simulink model "osservatore_con_fnc"  (R2024b)
settings: Solver=VariableStepAuto  StartTime=0.0  StopTime=10.0  RelTol=1e-3
values from neighbouring files (symbols this model uses):
  A4 = horzcat([0;0;0;0], A4)    [stabilita_AS.m]
  BB = [0; B]    [stabilita_AS.m]
  KK = [0 K]    [stabilita_AS.m]
undefined symbols (not defined in the file or in its folder): L_oss_theta
settings Model: Creator=costa  LastModifiedBy=costa

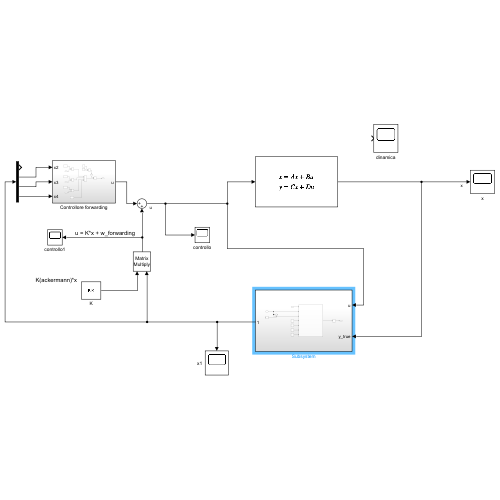
[thumbnail: Simulink's stored preview of the top-level diagram]
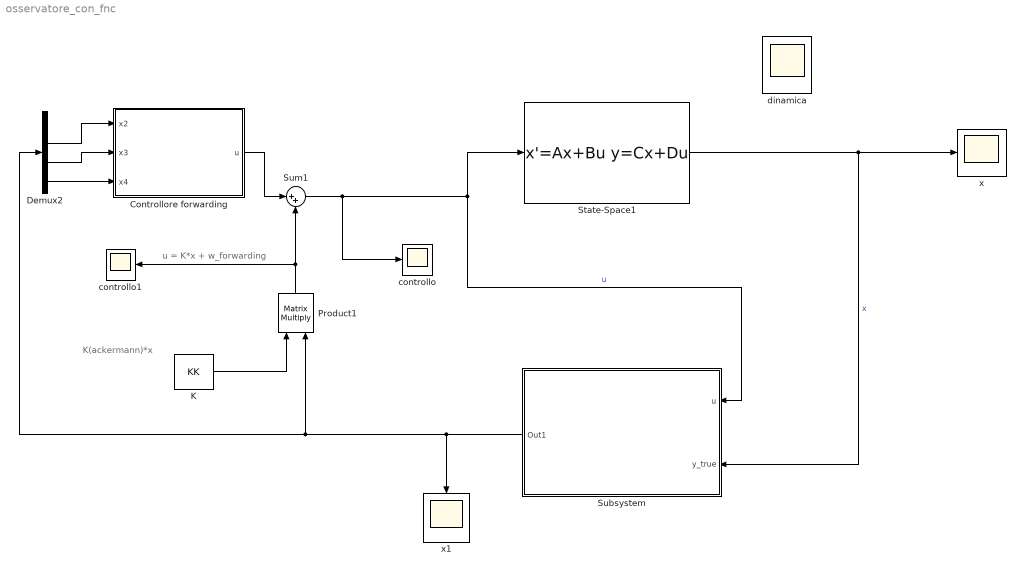
== system osservatore_con_fnc ==
  note: K(ackermann)*x
  note: u = K*x + w_forwarding
  Controllore forwarding : Subsystem
  Demux2 : Demux
  K : Constant  Value=KK  VectorParams1D=off
  Product1 : Product  Multiplication=Matrix(*)
  State-Space1 : StateSpace  A=A4  B=BB  C=eye(4)  D=[0; 0; 0; 0]  InitialCondition=[1 0 0 0]
  Subsystem : Subsystem
  Sum1 : Sum  Inputs=|++
  controllo : Scope
  controllo1 : Scope
  dinamica : Scope
  x : Scope
  x1 : Scope
  wires:
  K/1 -> Product1/1
  Sum1/1 -> controllo/1, State-Space1/1, Subsystem/1(u)  "u"
  State-Space1/1 -> Subsystem/2(y_true), x/1  "x"
  Product1/1 -> controllo1/1, Sum1/2
  Subsystem/1(Out1) -> Demux2/1, Product1/2, x1/1
  Demux2/2 -> Controllore forwarding/1(x2)
  Demux2/3 -> Controllore forwarding/2(x3)
  Demux2/4 -> Controllore forwarding/3(x4)
  Controllore forwarding/1(u) -> Sum1/1

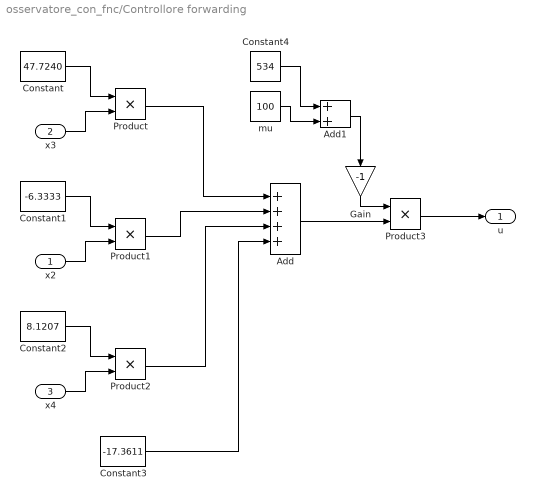
== system osservatore_con_fnc/Controllore forwarding ==
  x2 : Inport
  x3 : Inport  Port=2
  x4 : Inport  Port=3
  Add : Sum  Inputs=++++
  Add1 : Sum
  Constant : Constant  Value=47.7240
  Constant1 : Constant  Value=-6.3333
  Constant2 : Constant  Value=8.1207
  Constant3 : Constant  Value=-17.3611
  Constant4 : Constant  Value=534
  Gain : Gain  Gain=-1
  Product{,1..3} (4 alike) : Product
  mu : Constant  Value=100
  u : Outport
  wires:
  x3/1 -> Product/2
  Constant/1 -> Product/1
  Constant1/1 -> Product1/1
  x2/1 -> Product1/2
  Constant2/1 -> Product2/1
  x4/1 -> Product2/2
  Product/1 -> Add/1
  Product1/1 -> Add/2
  Product2/1 -> Add/3
  Constant3/1 -> Add/4
  Add/1 -> Product3/2
  Product3/1 -> u/1
  Constant4/1 -> Add1/1
  mu/1 -> Add1/2
  Add1/1 -> Gain/1
  Gain/1 -> Product3/1

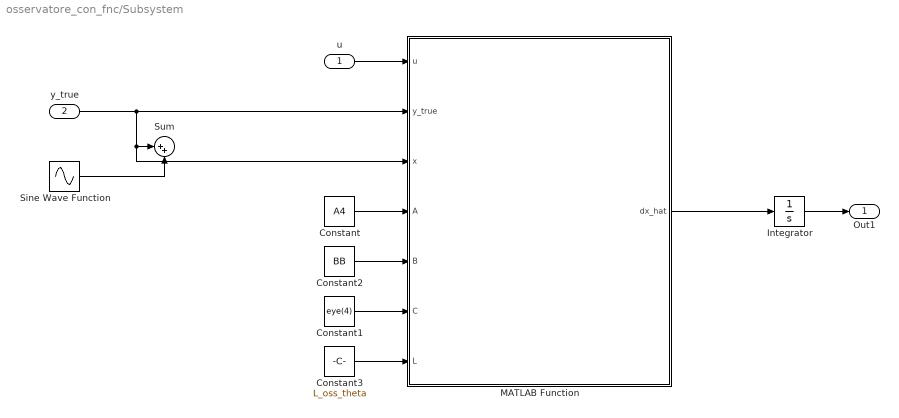
== system osservatore_con_fnc/Subsystem ==
  u : Inport
  y_true : Inport  Port=2
  Constant : Constant  Value=A4  VectorParams1D=off
  Constant1 : Constant  Value=eye(4)
  Constant2 : Constant  Value=BB
  Constant3 : Constant  Value=L_oss_theta  VectorParams1D=off
  Integrator : Integrator
  MATLAB Function : MATLAB Function  TreatAsAtomicUnit=on
  Sine Wave Function : Sin  TimeSource=Use external signal  Amplitude=0.1  Frequency=2*pi*50  SampleTime=0
  Sum : Sum  Inputs=|++
  Out1 : Outport
  wires:
  u/1 -> MATLAB Function/1(u)
  MATLAB Function/1(dx_hat) -> Integrator/1
  y_true/1 -> Sum/1, MATLAB Function/3(x), MATLAB Function/2(y_true)
  Integrator/1 -> Out1/1
  Constant1/1 -> MATLAB Function/6(C)
  Constant2/1 -> MATLAB Function/5(B)
  Constant/1 -> MATLAB Function/4(A)
  Constant3/1 -> MATLAB Function/7(L)
  Sine Wave Function/1 -> Sum/2

== matlab function osservatore_con_fnc/Subsystem/MATLAB Function ==
  data: u input; dx_hat output; y_true input; x input; A input; B input; C input; L input
function dx_hat = fcn(u, y_true, x, A, B, C, L)
    dx_hat = A*x + B*u + L*(y_true-C*x);
end
